simulink model "Stabilisation_trajectoire"  (R2025a)
settings: Solver=VariableStepAuto  StartTime=0.0  StopTime=20  RelTol=1e-3
libraries: dspmathops x1
settings Model: Creator=romai  LastModifiedBy=romai

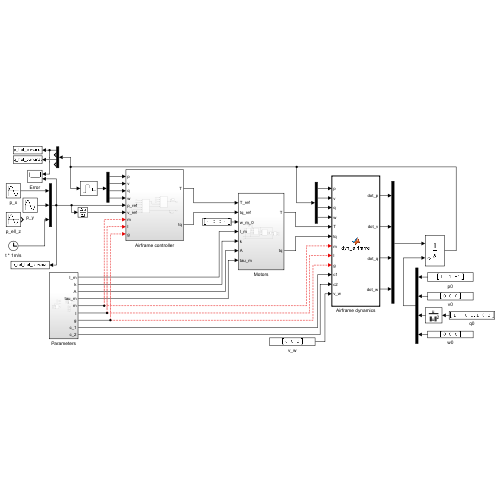
[thumbnail: Simulink's stored preview of the top-level diagram]
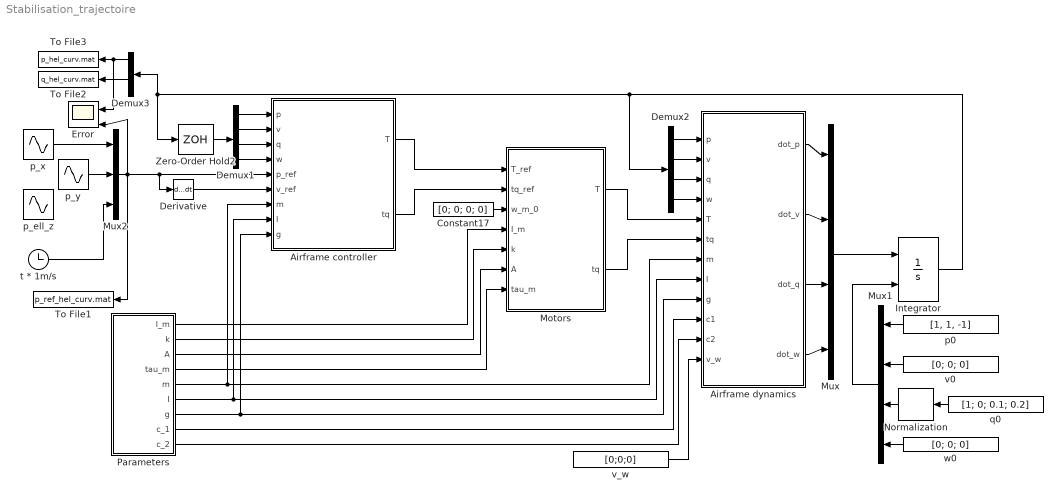
== system Stabilisation_trajectoire ==
  Airframe controller : Subsystem
  Airframe dynamics : MATLAB Function  TreatAsAtomicUnit=on
  Constant17 : Constant  Value=[0; 0; 0; 0]
  Demux1 : Demux  Outputs=[3, 3, 4, 3]
  Demux2 : Demux  Outputs=[3, 3, 4, 3]
  Demux3 : Demux  Outputs=[3, 3, 4, 3]
  Derivative : Derivative
  Error : Scope  NumInputPorts=2
      settings: ActiveDisplayYMinimum=-10.846311918162851  ActiveDisplayYMaximum=13.551571009977819
  Integrator : Integrator  InitialConditionSource=external
  Motors : Subsystem
  Mux : Mux
  Mux1 : Mux
  Mux2 : Mux  Inputs=3
  Normalization : dspmathops/Normalization  NormType=Squared 2-norm  Bias=1e-10  NormOver=Each column  Dimension=1  roundingMode=Floor  overflowMode=off  accumDataTypeStr=Inherit: Same as product output  accumLastDataTypeStr=Inherit: Same as product output  outputDataTypeStr=Inherit: Same as product output  outputMin=[]  outputMax=[]  outputLastDataTypeStr=Inherit: Same as product output
  Parameters : Subsystem
  To File1 : ToFile  Filename=p_ref_hel_curv.mat  SampleTime=0.05
  To File2 : ToFile  Filename=q_hel_curv.mat  SampleTime=0.05
  To File3 : ToFile  Filename=p_hel_curv.mat  SampleTime=0.05
  Zero-Order Hold2 : ZeroOrderHold  SampleTime=0.01
  p0 : Constant  Value=[1, 1, -1]
  p_ell_z : Sin  Frequency=0.5  Phase=2 * pi/3  SampleTime=0
  p_x : Sin  Amplitude=3  Frequency=4  Phase=pi/3  SampleTime=0
  p_y : Sin  Amplitude=3  Frequency=4  SampleTime=0
  q0 : Constant  Value=[1; 0; 0.1; 0.2]
  t * 1m/s : Clock
  v0 : Constant  Value=[0; 0; 0]
  v_w : Constant  Value=[0;0;0]
  w0 : Constant  Value=[0; 0; 0]
  wires:
  Mux1/1 -> Integrator/2
  Airframe dynamics/1(dot_p) -> Mux/1
  Demux2/2 -> Airframe dynamics/2(v)
  Mux/1 -> Integrator/1
  Airframe dynamics/2(dot_v) -> Mux/2
  Integrator/1 -> Demux2/1, Zero-Order Hold2/1, Demux3/1
  Demux2/4 -> Airframe dynamics/4(w)
  Demux1/1 -> Airframe controller/1(p)
  Demux1/4 -> Airframe controller/4(w)
  v0/1 -> Mux1/2
  p0/1 -> Mux1/1
  Demux1/2 -> Airframe controller/2(v)
  w0/1 -> Mux1/4
  Constant17/1 -> Motors/3(w_m_0)
  Airframe controller/1(T) -> Motors/1(T_ref)
  Parameters/1(I_m) -> Motors/4(I_m)
  Parameters/2(k) -> Motors/5(k)
  Parameters/3(A) -> Motors/6(A)
  Parameters/4(tau_m) -> Motors/7(tau_m)
  Parameters/5(m) -> Airframe controller/7(m), Airframe dynamics/7(m)
  Parameters/6(I) -> Airframe controller/8(I), Airframe dynamics/8(I)
  Parameters/7(g) -> Airframe controller/9(g), Airframe dynamics/9(g)
  Demux1/3 -> Airframe controller/3(q)
  Airframe dynamics/4(dot_w) -> Mux/4
  Normalization/1 -> Mux1/3
  v_w/1 -> Airframe dynamics/12(v_w)
  Parameters/8(c_1) -> Airframe dynamics/10(c1)
  Parameters/9(c_2) -> Airframe dynamics/11(c2)
  Mux2/1 -> To File1/1, Derivative/1, Airframe controller/5(p_ref), Error/2
  Demux2/1 -> Airframe dynamics/1(p)
  Derivative/1 -> Airframe controller/6(v_ref)
  Motors/1(T) -> Airframe dynamics/5(T)
  Motors/2(tq) -> Airframe dynamics/6(tq)
  Zero-Order Hold2/1 -> Demux1/1
  Airframe controller/2(tq) -> Motors/2(tq_ref)
  Demux2/3 -> Airframe dynamics/3(q)
  Airframe dynamics/3(dot_q) -> Mux/3
  q0/1 -> Normalization/1
  Demux3/1 -> Error/1, To File3/1
  Demux3/3 -> To File2/1
  t * 1m/s/1 -> Mux2/3
  p_x/1 -> Mux2/1
  p_y/1 -> Mux2/2

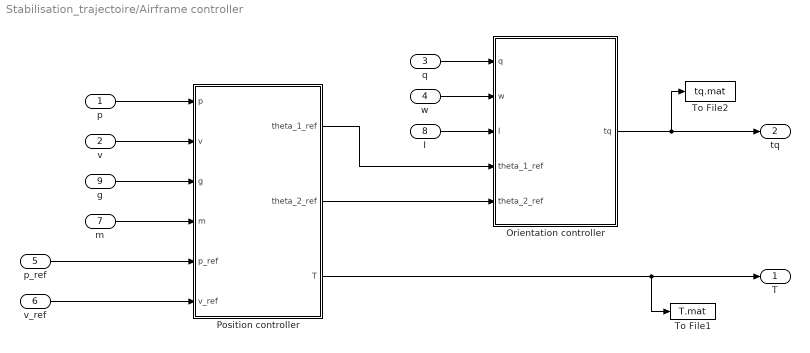
== system Stabilisation_trajectoire/Airframe controller ==
  p : Inport
  v : Inport  Port=2
  q : Inport  Port=3
  w : Inport  Port=4
  p_ref : Inport  Port=5
  v_ref : Inport  Port=6
  m : Inport  Port=7
  I : Inport  Port=8
  g : Inport  Port=9
  Orientation controller : MATLAB Function  TreatAsAtomicUnit=on
  Position controller : MATLAB Function  TreatAsAtomicUnit=on
  To File1 : ToFile  Filename=T.mat
  To File2 : ToFile  Filename=tq.mat
  T : Outport
  tq : Outport  Port=2
  wires:
  w/1 -> Orientation controller/2(w)
  g/1 -> Position controller/3(g)
  p/1 -> Position controller/1(p)
  v/1 -> Position controller/2(v)
  I/1 -> Orientation controller/3(I)
  Orientation controller/1(tq) -> tq/1, To File2/1
  Position controller/1(theta_1_ref) -> Orientation controller/4(theta_1_ref)
  Position controller/2(theta_2_ref) -> Orientation controller/5(theta_2_ref)
  Position controller/3(T) -> T/1, To File1/1
  m/1 -> Position controller/4(m)
  q/1 -> Orientation controller/1(q)
  v_ref/1 -> Position controller/6(v_ref)
  p_ref/1 -> Position controller/5(p_ref)

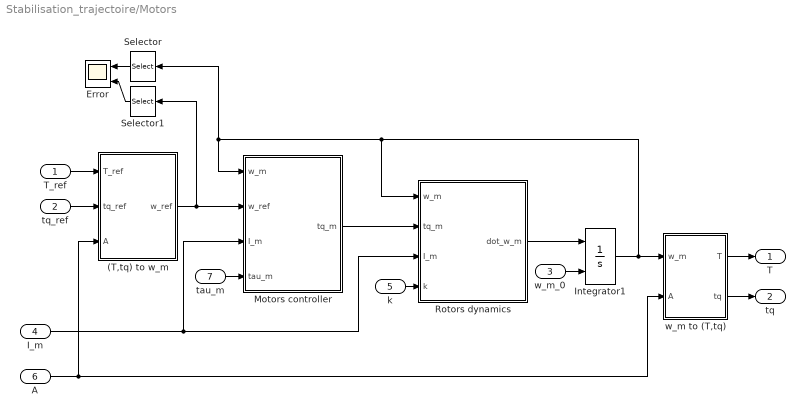
== system Stabilisation_trajectoire/Motors ==
  T_ref : Inport
  tq_ref : Inport  Port=2
  w_m_0 : Inport  Port=3
  I_m : Inport  Port=4
  k : Inport  Port=5
  A : Inport  Port=6
  tau_m : Inport  Port=7
  (T,tq) to w_m : MATLAB Function  TreatAsAtomicUnit=on
  Error : Scope  NumInputPorts=2
      settings: ActiveDisplayYMinimum=-2016.735931138054  ActiveDisplayYMaximum=224.08177012645038
  Integrator1 : Integrator  InitialConditionSource=external
  Motors controller : MATLAB Function  TreatAsAtomicUnit=on
  Rotors dynamics : MATLAB Function  TreatAsAtomicUnit=on
  Selector : Selector  InputPortWidth=4  IndexOptions=Index vector (dialog)  Indices=1  OutputSizes=1
  Selector1 : Selector  InputPortWidth=4  IndexOptions=Index vector (dialog)  Indices=1  OutputSizes=1
  w_m to (T,tq) : MATLAB Function  TreatAsAtomicUnit=on
  T : Outport
  tq : Outport  Port=2
  wires:
  Rotors dynamics/1(dot_w_m) -> Integrator1/1
  Motors controller/1(tq_m) -> Rotors dynamics/2(tq_m)
  (T,tq) to w_m/1(w_ref) -> Selector1/1, Motors controller/2(w_ref)
  tq_ref/1 -> (T,tq) to w_m/2(tq_ref)
  A/1 -> w_m to (T,tq)/2(A), (T,tq) to w_m/3(A)
  Integrator1/1 -> Rotors dynamics/1(w_m), Motors controller/1(w_m), Selector/1, w_m to (T,tq)/1(w_m)
  T_ref/1 -> (T,tq) to w_m/1(T_ref)
  I_m/1 -> Rotors dynamics/3(I_m), Motors controller/3(I_m)
  tau_m/1 -> Motors controller/4(tau_m)
  w_m to (T,tq)/2(tq) -> tq/1
  w_m to (T,tq)/1(T) -> T/1
  w_m_0/1 -> Integrator1/2
  k/1 -> Rotors dynamics/4(k)
  Selector/1 -> Error/1
  Selector1/1 -> Error/2

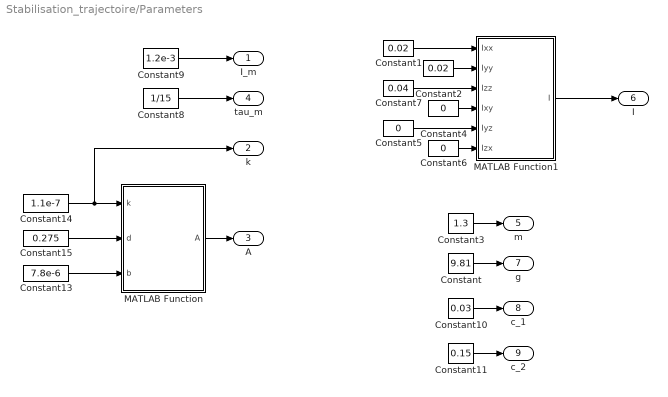
== system Stabilisation_trajectoire/Parameters ==
  Constant : Constant  Value=9.81
  Constant1 : Constant  Value=0.02
  Constant10 : Constant  Value=0.03
  Constant11 : Constant  Value=0.15
  Constant13 : Constant  Value=7.8e-6
  Constant14 : Constant  Value=1.1e-7
  Constant15 : Constant  Value=0.275
  Constant2 : Constant  Value=0.02
  Constant3 : Constant  Value=1.3
  Constant4 : Constant  Value=0
  Constant5 : Constant  Value=0
  Constant6 : Constant  Value=0
  Constant7 : Constant  Value=0.04
  Constant8 : Constant  Value=1/15
  Constant9 : Constant  Value=1.2e-3
  MATLAB Function : MATLAB Function  TreatAsAtomicUnit=on
  MATLAB Function1 : MATLAB Function  TreatAsAtomicUnit=on
  I_m : Outport
  k : Outport  Port=2
  A : Outport  Port=3
  tau_m : Outport  Port=4
  m : Outport  Port=5
  I : Outport  Port=6
  g : Outport  Port=7
  c_1 : Outport  Port=8
  c_2 : Outport  Port=9
  wires:
  Constant2/1 -> MATLAB Function1/2(Iyy)
  Constant5/1 -> MATLAB Function1/5(Iyz)
  Constant4/1 -> MATLAB Function1/4(Ixy)
  Constant7/1 -> MATLAB Function1/3(Izz)
  Constant1/1 -> MATLAB Function1/1(Ixx)
  Constant15/1 -> MATLAB Function/2(d)
  Constant6/1 -> MATLAB Function1/6(Izx)
  Constant13/1 -> MATLAB Function/3(b)
  MATLAB Function/1(A) -> A/1
  Constant8/1 -> tau_m/1
  Constant3/1 -> m/1
  Constant/1 -> g/1
  MATLAB Function1/1(I) -> I/1
  Constant9/1 -> I_m/1
  Constant14/1 -> MATLAB Function/1(k), k/1
  Constant10/1 -> c_1/1
  Constant11/1 -> c_2/1

== matlab function Stabilisation_trajectoire/Motors/Rotors dynamics ==
  data: w_m input; tq_m input; I_m input; dot_w_m output; k input
function dot_w_m  = dyn_rotors(w_m, tq_m, I_m, k)
    % Compute the time derivative of the angular velocities of the 4 rotors.
    %
    % Inputs:
    %   w_m    [4x1] Angular velocities of the 4 rotors.
    %   tq_m   [4x1] Torques generated by the 4 motors.
    %   I_m    [1x1] Single rotor (+ propeller?) rotational inertia with respect to its axis of rotation.
    %   k      [1x1] Drag parameter.
    %
    % Outputs:
    %   dot_w_m  [4x1] Time derivative of the angular velocities of the 4 rotors.

    drag = k * w_m .* abs(w_m);
    dot_w_m = (tq_m - drag) / I_m;
end

== matlab function Stabilisation_trajectoire/Motors/w_m to (T,tq) ==
  data: w_m input; T output; tq output; A input
function [T, tq] = fcn(w_m, A)
    w_squared = w_m.^2;
    T = A(1,:) * w_squared;
    tq = A(2:4,:) * w_squared;
end

== matlab function Stabilisation_trajectoire/Airframe controller/Orientation controller ==
  data: q input; tq output; w input; I input; theta_1_ref input; theta_2_ref input
function tq  = control_acc(q, w, I, theta_1_ref, theta_2_ref)
    qv = q(2:4);
    
    k_theta=100;
    k_omega=20;
    
    tq_x = I(1,1) * (-k_theta * (2*qv(1) - theta_1_ref) - k_omega * (w(1) ));
    tq_y = I(2,2) * (-k_theta * (2*qv(2) - theta_2_ref) - k_omega * (w(2) ));
    tq_z = I(3,3) * (-k_theta * (2*qv(3)) - k_omega * (w(3) ));
    tq = [tq_x; tq_y; tq_z];

end

== matlab function Stabilisation_trajectoire/Airframe controller/Position controller ==
  data: theta_1_ref output; theta_2_ref output; p input; v input; g input; m input; p_ref input; T output; v_ref input
function [theta_1_ref, theta_2_ref, T] = control_pos(p,v,g,m,p_ref, v_ref) 
    k_p = 4;
    k_v = 4;

    theta_2_ref = (-1/g) * (-k_p * (p(1) - p_ref(1)) - k_v * (v(1)- v_ref(1)));

    theta_1_ref = (1 / g) * (-k_p * (p(2) - p_ref(2)) - k_v * (v(2)-v_ref(2)));
    
    T = m * g + m*(1 * (p(3) - p_ref(3)) + 2 * (v(3) - v_ref(3)));
end

== matlab function Stabilisation_trajectoire/Airframe dynamics ==
  data: p input; v input; dot_p output; dot_v output; q input; w input; T input; tq input; m input; I input; g input; c1 input; c2 input; dot_q output; dot_w output; v_w input
function [dot_p, dot_v, dot_q, dot_w] = dyn_airframe(p,v,q,w, T,tq, m,I,g,c1,c2,v_w)

    % Compute the time derivative of the state (p,v,q,w) of the drone's airframe, neglecting
    % the gyroscopic effects induced by the propellers.
    %
    % Inputs:
    %  - State variables:
    %   p       [3x1] Position.
    %   v       [3x1] Velocity.
    %   q       [4x1] Orientation to be interpreted as a unit quaternion (simulink doesn't support quaternion signals).
    %   w       [3x1] Angular velocity (in the drone's frame).
    %
    %  - Control variables:
    %   T       [1x1] Thrust generated by the 4 propellers.
    %   tq      [3x1] Torque generated by the 4 propellers (in the drone's frame).
    %
    %  - Constant parameters:
    %   m       [1x1] Mass of the drone.
    %   I       [3x3] Rotational inertia matrix of the drone (in the drone's frame).
    %   g       [1x1] Gravitational acceleration (positive).
    %
    % Outputs:
    %   dot_p   [3x1] Time derivative of position.
    %   dot_v   [3x1] Time derivative of velocity.
    %   dot_q   [4x1] Time derivative of orientation to be interpreted as a quaternion in T_q(S^3).
    %   dot_w   [3x1] Time derivative of angular velocity.
    
    q = quaternion(q');
  
    % Airframe drift
    v_a = v - v_w;
    D = norm(v_a) * rotatepoint(q, [c1,c1,c2] .* rotatepoint(conj(q), v_a'))';
    
    dot_p = v;
    dot_v = [0;0;g] - T/m * rotatepoint(q, [0,0,1])' - D;
    dot_q = compact(q * quaternion([0, w'/2]) - (norm(q)^2 - 1) * q)';
    dot_w = I \ (tq - cross(w, I * w));
end

== matlab function Stabilisation_trajectoire/Parameters/MATLAB Function ==
  data: k input; d input; b input; A output
function A = fcn(k,d,b)
    
    db = d*b;

    A = [ b    b    b    b;
          0   db    0  -db;
         db    0  -db    0;
          k   -k    k   -k ];
end

== matlab function Stabilisation_trajectoire/Parameters/MATLAB Function1 ==
  data: Ixx input; I output; Iyy input; Izz input; Ixy input; Iyz input; Izx input
function I = fcn(Ixx, Iyy, Izz, Ixy, Iyz, Izx)
    
    I = [Ixx  Ixy  Izx;
         Ixy  Iyy  Iyz;
         Izx  Iyz  Izz];
end

== matlab function Stabilisation_trajectoire/Motors/(T,tq) to w_m ==
  data: T_ref input; w_ref output; tq_ref input; A input
function w_ref = fcn(T_ref, tq_ref, A)
    w_squared = A \ [T_ref; tq_ref];
    w_squared(w_squared < 0) = 0;
    w_ref = sqrt(w_squared) .* [-1; 1; -1; 1];
end

== matlab function Stabilisation_trajectoire/Motors/Motors controller ==
  data: w_m input; w_ref input; tq_m output; I_m input; tau_m input
function tq_m = ESC(w_m, w_ref, I_m, tau_m)  % dot_wref ?
    tq_m = I_m * (-1/tau_m) * (w_m - w_ref);
end
